simulink model "wo_switch"  (R2016a)
settings: Solver=VariableStepAuto  StartTime=0.0  StopTime=0.3  RelTol=1e-3
values from neighbouring files (symbols this model uses):
  duty_cycle = duty_cycle + temp    (= 1)    [teng_functions.m]
libraries: powerlib x17, powerlib_meascontrol x1, simulink x1
settings Model: Creator=user  LastModifiedBy=mugino

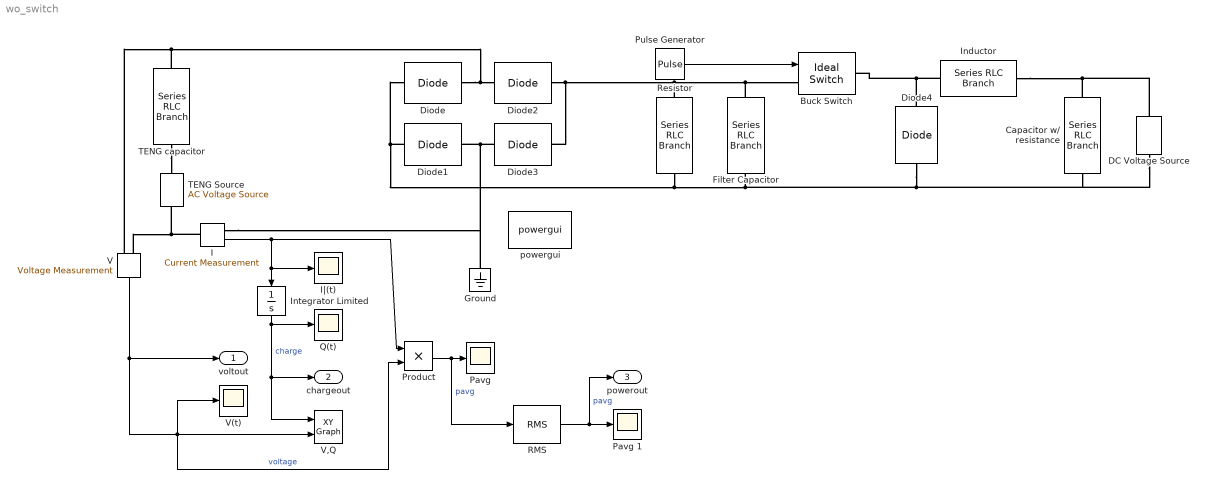
== system wo_switch ==
  Buck Switch : powerlib/Power Electronics/Ideal Switch  Ron=0.001  Lon=0  IC=0  Rs=1e5  Cs=inf  Measurements=off
  Capacitor w/ resistance : powerlib/Elements/Series RLC Branch  LConnTagsString=__new0  RConnTagsString=__new0  BranchType=RC  Resistance=100  Inductance=1e-3  SetiL0=off  InitialCurrent=0  Capacitance=10e-4  Setx0=off  InitialVoltage=0  Measurements=None
  DC Voltage Source : powerlib/Electrical Sources/DC Voltage Source  Amplitude=300  Measurements=None
  Diode{,1..3} (4 alike) : powerlib/Power Electronics/Diode  Ron=0.001  Lon=1e-3  Vf=0.5  IC=0  UseSnubber=off  Rs=500  Cs=250e-9  Measurements=off
  Diode4 : powerlib/Power Electronics/Diode  Ron=0.001  Lon=0  Vf=0.7  IC=0  UseSnubber=off  Rs=500  Cs=250e-9  Measurements=off
  Filter Capacitor : powerlib/Elements/Series RLC Branch  LConnTagsString=__new0  RConnTagsString=__new0  BranchType=C  Resistance=10  Inductance=1e-3  SetiL0=off  InitialCurrent=0  Capacitance=10e-5  Setx0=off  InitialVoltage=0  Measurements=None
  Ground : powerlib/Elements/Ground  LConnTagsString=a
  I : powerlib/Measurements/Current Measurement  PhasorSimulation=off  OutputType=Complex  PSBequivalent=0
  Inductor : powerlib/Elements/Series RLC Branch  LConnTagsString=__new0  RConnTagsString=__new0  BranchType=L  Resistance=0  Inductance=2  SetiL0=off  InitialCurrent=0  Capacitance=0  Setx0=off  InitialVoltage=0  Measurements=None
  Integrator Limited : Integrator  LimitOutput=on  UpperSaturationLimit=1  LowerSaturationLimit=0
  I|(t) : Scope
  "Pavg " : Scope
  Pavg 1 : Scope
  Product : Product
  Pulse Generator : DiscretePulseGenerator  PulseType=Time based  Period=5e-5  PulseWidth=duty_cycle
  Q(t) : Scope
  RMS : powerlib_meascontrol/Measurements/RMS  TrueRMS=on  Freq=50  RMSInit=0  Ts=0
  Resistor : powerlib/Elements/Series RLC Branch  LConnTagsString=__new0  RConnTagsString=__new0  BranchType=R  Resistance=500  Inductance=1e-3  SetiL0=off  InitialCurrent=0  Capacitance=10e-5  Setx0=off  InitialVoltage=0  Measurements=None
  TENG Source : powerlib/Electrical Sources/AC Voltage Source  Amplitude=310  Phase=0  Frequency=50  SampleTime=0  Measurements=None  BusType=PV  Pref=10e3  Qref=0  Qmin=-inf  Qmax=+inf
  TENG capacitor : powerlib/Elements/Series RLC Branch  LConnTagsString=__new0  RConnTagsString=__new0  BranchType=RC  Resistance=1000  Inductance=1e-3  SetiL0=off  InitialCurrent=0  Capacitance=9e-7  Setx0=off  InitialVoltage=0  Measurements=None
  V : powerlib/Measurements/Voltage Measurement  PhasorSimulation=off  OutputType=Complex  PSBequivalent=0
  V(t) : Scope
  V,Q : simulink/Sinks/XY Graph  xmin=-1e-6  xmax=5.5e-4  ymin=-300  ymax=300  st=-1
  powergui : powerlib/powergui  Priority=1  SimulationMode=Continuous  SolverType=Tustin/Backward Euler (TBE)  SampleTime=50e-6  frequency=60  SPID=on  DisableSnubberDevices=off  DisableRonSwitches=off  DisableVfSwitches=off  SwTol=0  DisplayEquations=off  Interpol=off  ExternalGateDelay=off  methode=off  Ts=10  FunctionMessages=off  echomessages=off  HookPort=off  EnableUseOfTLC=off  x0status=steady  frequencyindice=0  Pbase=100e6  ErrMax=1e-4  Iterations=50  UnitsV=kV  UnitsW=MW  buscounter=0  RestoreLinks=warning  ResistiveCurrentMeasurement=off  Frange=[0:2:500]  Ylog=off  Xlog=on  ShowGrid=off  save=off  variable=ZData  structure=0  ZoomFFT=off  StartTime=0.0  cycles=1  DisplayStyle=1  fundamental=60  FreqAxis=off  MaxFrequency=1000  frequencyindicesteady=1  RmsSteady=1  display=off
  voltout : Outport
  chargeout : Outport  Port=2
  powerout : Outport  Port=3
  wires:
  Integrator Limited/1 -> chargeout/1, V,Q/1, Q(t)/1  "charge"
  Pulse Generator/1 -> Buck Switch/1
  V/1 -> V(t)/1, V,Q/2, Product/2, voltout/1  "voltage"
  I/1 -> Product/1, I|(t)/1, Integrator Limited/1
  Product/1 -> RMS/1, "Pavg "/1  "pavg"
  RMS/1 -> powerout/1, Pavg 1/1  "pavg"
  connections:
  TENG capacitor/LConn1 -- V/LConn1 -- Diode2/LConn1 -- Diode/RConn1
  Diode3/LConn1 -- I/RConn1 -- Ground/LConn1 -- Diode1/RConn1
  V/LConn2 -- I/LConn1 -- TENG Source/LConn1
  TENG capacitor/RConn1 -- TENG Source/RConn1
  DC Voltage Source/RConn1 -- Inductor/RConn1 -- Capacitor w/ resistance/LConn1
  Diode1/LConn1 -- Diode4/LConn1 -- DC Voltage Source/LConn1 -- Capacitor w/ resistance/RConn1 -- Filter Capacitor/RConn1 -- Resistor/RConn1 -- Diode/LConn1
  Diode2/RConn1 -- Diode3/RConn1 -- Buck Switch/LConn1 -- Filter Capacitor/LConn1 -- Resistor/LConn1
  Inductor/LConn1 -- Diode4/RConn1 -- Buck Switch/RConn1
